simulink model "main_RI_LIEKF_GNSSOutrage"  (R2023a)
settings: Solver=FixedStepAuto  StartTime=0.0  StopTime=220  FixedStep=0.01  RelTol=1e-3
InitFcn:
  | initNavigation0612_AOA;
values from neighbouring files (symbols this model uses):
  CF_enable = 0    [initNavigation.m]
  dt = 0.01    [initNavigation.m]
  dtDelay = -0.03    [initNavigation.m]
  g0 = 9.795    [initNavigation.m]
  gam0_rad = 0/57.3    (= 0)    [initNavigation.m]
  GNSSoutragetime = 90    [initNavigation.m]
  H_sensor_type = 0    [initNavigation.m]
  KF_enable = 1    [initNavigation.m]
  P0 = diag([1*ones(3,1);0.01*ones(3,1);0.1*ones(3,1);0.001*ones(3,1);0.00001*ones(3,1)])    [initNavigation.m]
  P0_RIEKF = diag([1*ones(3,1);0.01*ones(3,1);0.1*ones(3,1);0.001*ones(3,1);0.00001*ones(3,1);      0.01*ones(3,1);[0;2;2]/57.3;[0.1;0.1;0.1]])^2    [initNavigation.m]
  pd0 = 0    [initNavigation.m]
  pe0 = 0    [initNavigation.m]
  phi0_rad = 0/57.3    (= 0)    [initNavigation.m]
  pn0 = 0    [initNavigation.m]
  psi = -178    [initNavigation.m]
  psi0_rad = 0/57.3    (= 0)    [initNavigation.m]
  state_dim = 24    [initNavigation.m]
  Time = 0:0.01:(size(traindata.AttackAngle,1) - 1)*0.01    [NNLiftCoefficientFit.m]
  vd0 = 0    [initNavigation.m]
  ve0 = 0    [initNavigation.m]
  vn0 = 0    [initNavigation.m]
undefined symbols (not defined in the file or in its folder): DiscIntNeverNeededParam, Discrete, INS_CONST, INS_EXPORT, INS_PARAM, magnitude, p, param, pInitialization, sys
libraries: simulink_extras x94, simulink x82, dspstat3 x70, sharedtransform x60, ctrlSharedLib x36, sharedTrackingLibrary x22, matrix_library x15, FMT_Model_Lib x13, deeplib x8, dspsolvers x4, vrlib x4, aerolibconvert2 x1
(part 17 of 28)

== system main_RI_LIEKF_GNSSOutrage/State estimation/LI EKF2/INS propogation/vel//pos update/vel update ==
  dtheta : Inport
  QGC_init : Inport  Port=2
  An : Inport  Port=3
  KFState_dv : Inport  Port=4
  v0 : Inport  Port=5
  Cbn : Inport  Port=6
  Add : Sum
  Delay : Delay  DelayLength=1  InitialConditionSource=Input port  ExternalReset=Rising
      settings: InputPortMap=u0,r5,p4
  Gain : Gain  Gain=dt
  MATLAB Function : MATLAB Function  TreatAsAtomicUnit=on
  Reshape : Reshape  OutputDimensionality=Column vector (2-D)
  vel_k : Outport
  wires:
  Cbn/1 -> MATLAB Function/4(Cbn)
  QGC_init/1 -> Delay/2
  Reshape/1 -> Delay/3
  An/1 -> Gain/1
  v0/1 -> Reshape/1
  Gain/1 -> Add/1
  Delay/1 -> Add/2
  KFState_dv/1 -> MATLAB Function/2(KFState_dv)
  dtheta/1 -> MATLAB Function/1(dtheta)
  Add/1 -> MATLAB Function/3(vel)
  MATLAB Function/1(vel_correct) -> Delay/1, vel_k/1

== system main_RI_LIEKF_GNSSOutrage/State estimation/RI EKF_AOA_LSTM/Error State Kalman Filter/Extended Kalman Filter1/Correct1 ==
  yMeas : Inport  SampleTime=SampleTime
  R : Inport  Port=2  SampleTime=SampleTime
  uMeas : Inport  Port=3  SampleTime=SampleTime
  uBlockOrdering : Inport  Port=4  SampleTime=SampleTime
  Enable : EnablePort
  Correct : MATLAB Function  TreatAsAtomicUnit=on
  Data Store ReadP : DataStoreRead  DataStoreName=P  IndexOptions=Index vector (dialog)  Indices=1  OutputSizes=1
  Data Store ReadX : DataStoreRead  DataStoreName=x  IndexOptions=Index vector (dialog)  Indices=1  OutputSizes=1
  Data Store WriteP : DataStoreWrite  DataStoreName=P  IndexOptions=Index vector (dialog)  Indices=1  OutputSizes=1
  Data Store WriteX : DataStoreWrite  DataStoreName=x  IndexOptions=Index vector (dialog)  Indices=1  OutputSizes=1
  IGG_check : Subsystem  Commented=on
  R1 : InportShadow  Port=2  SampleTime=SampleTime
  RegisterSimulinkFcn : S-Function  FunctionName=ekfukfRegisterSimulinkFcn  Parameters=int32(3), 1, pM.HasAdditiveNoise, SampleTime, DataType, SLFcnsToRegister  SFunctionDeploymentMode=off  EnableBusSupport=off
  Scope : Scope
  Scope1 : Scope
  Scope2 : Scope
  yMeas1 : InportShadow  SampleTime=SampleTime
  yBlockOrdering : Outport  VectorParamsAs1DForOutWhenUnconnected=off
  wires:
  uMeas/1 -> Correct/5(uMeas)
  uBlockOrdering/1 -> Correct/6("blockOrdering ")
  Correct/3(blockOrdering) -> yBlockOrdering/1
  Correct/1(xNew) -> Data Store WriteX/1
  R/1 -> RegisterSimulinkFcn/3, Correct/4(R)
  yMeas/1 -> Scope/1, RegisterSimulinkFcn/2, Correct/3(yMeas)
  Correct/2(P) -> Data Store WriteP/1
  Data Store ReadP/1 -> IGG_check/1(Pk/k_1), Correct/2("P ")
  yMeas1/1 -> IGG_check/2(yMeas)
  R1/1 -> IGG_check/4(R)
  IGG_check/2(w) -> Scope1/1
  Data Store ReadX/1 -> IGG_check/3(X), Correct/1(x), RegisterSimulinkFcn/1
  IGG_check/3(inno) -> Scope2/1

== system main_RI_LIEKF_GNSSOutrage/State estimation/RI EKF_AOA_LSTM/Error State Kalman Filter/Extended Kalman Filter1/Output ==
  uBlockOrdering : Inport
  Data Store Read : DataStoreRead  DataStoreName=x  IndexOptions=Index vector (dialog)  Indices=1  OutputSizes=1
  Data Store Read1 : DataStoreRead  DataStoreName=P  IndexOptions=Index vector (dialog)  Indices=1  OutputSizes=1
  MATLAB Function : MATLAB Function  TreatAsAtomicUnit=on
  x : Outport  VectorParamsAs1DForOutWhenUnconnected=off
  P : Outport  Port=2  VectorParamsAs1DForOutWhenUnconnected=off
  yBlockOrdering : Outport  Port=3  VectorParamsAs1DForOutWhenUnconnected=off
  wires:
  MATLAB Function/1(P) -> P/1
  uBlockOrdering/1 -> yBlockOrdering/1
  Data Store Read1/1 -> MATLAB Function/1(S)
  Data Store Read/1 -> x/1

== system main_RI_LIEKF_GNSSOutrage/State estimation/RI EKF_AOA_LSTM/Error State Kalman Filter/Extended Kalman Filter1/Predict ==
  Q : Inport  SampleTime=SampleTime
  uState : Inport  Port=2  SampleTime=SampleTime
  uBlockOrdering : Inport  Port=3  SampleTime=SampleTime
  Data Store Read1 : DataStoreRead  Commented=on  DataStoreName=feedback_flag_18dim  IndexOptions=Index vector (dialog)  Indices=1  OutputSizes=1
  Data Store Write : DataStoreWrite  DataStoreName=P  IndexOptions=Index vector (dialog)  Indices=1  OutputSizes=1
  Data Store Write1 : DataStoreWrite  DataStoreName=x  IndexOptions=Index vector (dialog)  Indices=1  OutputSizes=1
  Data Store WriteX : DataStoreWrite  DataStoreName=x  IndexOptions=Index vector (dialog)  Indices=1  OutputSizes=1
  Data Store ReadP : DataStoreRead  DataStoreName=P  IndexOptions=Index vector (dialog)  Indices=1  OutputSizes=1
  Data Store ReadX : DataStoreRead  DataStoreName=x  IndexOptions=Index vector (dialog)  Indices=1  OutputSizes=1
  If : If  Commented=on  IfExpression=u1 == 1  ShowElse=off
  If Action Subsystem : Subsystem  Commented=on  TreatAsAtomicUnit=on
  Predict : MATLAB Function  TreatAsAtomicUnit=on
  RegisterSimulinkFcn : S-Function  FunctionName=ekfukfRegisterSimulinkFcn  Parameters=int32(2), 0, pS.HasAdditiveNoise, SampleTime, DataType, SLFcnsToRegister  SFunctionDeploymentMode=off  EnableBusSupport=off
  Zero : Constant  Value=zeros(state_dim,1)  OutDataTypeStr=Inherit: Inherit via back propagation
  wires:
  Zero/1 -> Data Store Write1/1
  If/1 -> If Action Subsystem/Action
  Data Store Read1/1 -> If/1
  uState/1 -> Predict/4(uState)
  uBlockOrdering/1 -> Predict/5(unused)
  Data Store ReadX/1 -> RegisterSimulinkFcn/1, Predict/1(x)
  Predict/1(xNew) -> Data Store WriteX/1
  Q/1 -> RegisterSimulinkFcn/2, Predict/3(Q)
  Predict/2(P) -> Data Store Write/1
  Data Store ReadP/1 -> Predict/2("P ")

== system main_RI_LIEKF_GNSSOutrage/State estimation/RI EKF_AOA_LSTM/Error State Kalman Filter/Simulink Function - State Transition/Cal Phi ==
  Rbn : Inport
  vn : Inport  Port=2
  pn : Inport  Port=3
  Constant : Constant  Value=dt
  MATLAB Function1 : MATLAB Function  TreatAsAtomicUnit=on
  Reshape : Reshape  OutputDimensionality=Column vector (2-D)
  Reshape1 : Reshape  OutputDimensionality=Column vector (2-D)
  Phi : Outport
  wires:
  Constant/1 -> MATLAB Function1/4(dt)
  MATLAB Function1/1(Phi) -> Phi/1
  Rbn/1 -> MATLAB Function1/3(Rbn)
  vn/1 -> Reshape/1
  pn/1 -> Reshape1/1
  Reshape/1 -> MATLAB Function1/1(vn)
  Reshape1/1 -> MATLAB Function1/2(pn)

== system main_RI_LIEKF_GNSSOutrage/State estimation/RI EKF_AOA_LSTM/Error State Kalman Filter/Simulink Function - State Transition1/Cal Phi ==
  Rbn : Inport
  vn : Inport  Port=2
  pn : Inport  Port=3
  Constant : Constant  Value=dt  OutDataTypeStr=single
  MATLAB Function1 : MATLAB Function  TreatAsAtomicUnit=on
  Reshape : Reshape  OutputDimensionality=Column vector (2-D)
  Reshape1 : Reshape  OutputDimensionality=Column vector (2-D)
  Phi : Outport
  wires:
  Reshape1/1 -> MATLAB Function1/2(pn)
  Reshape/1 -> MATLAB Function1/1(vn)
  pn/1 -> Reshape1/1
  vn/1 -> Reshape/1
  Rbn/1 -> MATLAB Function1/3(Rbn)
  MATLAB Function1/1(Phi) -> Phi/1
  Constant/1 -> MATLAB Function1/4(dt)

== system main_RI_LIEKF_GNSSOutrage/State estimation/RI EKF_AOA_LSTM/Error State Kalman Filter/bak/Simulink Function - GPS Measurements1 ==
  DCM_b_n : Inport
  DynamicMeasurementFcn_Dyn : TriggerPort  TriggerType=function-call  IsSimulinkFunction=on  FunctionName=DynamicMeasurementFcn_Dyn  VariantControl=Variant
  Add : Sum  Commented=on
  Add1 : Sum
  Constant : Constant  Commented=on  Value=dt  OutDataTypeStr=single
  Constant6 : Constant  Value=[zeros(3,3),eye(3),zeros(3,12);zeros(3,15),eye(3)]  OutDataTypeStr=single
  Data Type Conversion6 : DataTypeConversion  Commented=on  OutDataTypeStr=single  SaturateOnIntegerOverflow=off  RndMeth=Floor
  From7 : From  Commented=on  GotoTag=DCM_b_n
  Goto : Goto  Commented=on  GotoTag=DCM_b_n
  MATLAB Function1 : MATLAB Function  Commented=on  TreatAsAtomicUnit=on
  Product : Product  Commented=on  Multiplication=Matrix(*)
  Product1 : Product  Multiplication=Matrix(*)
  x : ArgIn  DisableCoverage=on  OutDataTypeStr=single  PortDimensions=18  ArgumentName=x
  v : ArgIn  DisableCoverage=on  Port=2  OutDataTypeStr=single  PortDimensions=6  ArgumentName=v
  y : ArgOut  DisableCoverage=on  OutDataTypeStr=single  PortDimensions=6  ArgumentName=y
  wires:
  Product/1 -> Add/1
  MATLAB Function1/1(H) -> Data Type Conversion6/1
  From7/1 -> MATLAB Function1/1(Cbn)
  Constant/1 -> MATLAB Function1/2(dt)
  DCM_b_n/1 -> Goto/1
  Data Type Conversion6/1 -> Product/1
  Add1/1 -> y/1
  v/1 -> Add1/2
  Product1/1 -> Add1/1
  Constant6/1 -> Product1/1
  x/1 -> Product1/2

== system main_RI_LIEKF_GNSSOutrage/State estimation/RI EKF_AOA_LSTM/Error State Kalman Filter/bak/Simulink Function - GPS Measurements2 ==
  ZUPTMeasurementFcn2 : TriggerPort  TriggerType=function-call  IsSimulinkFunction=on  FunctionName=ZUPTMeasurementFcn2  VariantControl=Variant
  Add : Sum
  Constant6 : Constant  Value=[zeros(3,3),eye(3),zeros(3,12)]  OutDataTypeStr=single
  Product : Product  Multiplication=Matrix(*)
  x : ArgIn  DisableCoverage=on  OutDataTypeStr=single  PortDimensions=18  ArgumentName=x
  v : ArgIn  DisableCoverage=on  Port=2  OutDataTypeStr=single  PortDimensions=3  ArgumentName=v
  y : ArgOut  DisableCoverage=on  OutDataTypeStr=single  PortDimensions=3  ArgumentName=y
  wires:
  Add/1 -> y/1
  Product/1 -> Add/1
  x/1 -> Product/2
  Constant6/1 -> Product/1
  v/1 -> Add/2

== system main_RI_LIEKF_GNSSOutrage/State estimation/RI EKF_AOA_LSTM/Error State Kalman Filter/bak/Simulink Function - State Transition Jacobian ==
  DCM_b_n : Inport
  vn : Inport  Port=2
  pn : Inport  Port=3
  stateTransitionJacobianFcn_Dyn : TriggerPort  TriggerType=function-call  IsSimulinkFunction=on  FunctionName=stateTransitionJacobianFcn_Dyn  VariantControl=Variant
  Cal Phi1 : Subsystem
  Constant : Constant  Value=0.01  OutDataTypeStr=single
  Data Type Conversion1 : DataTypeConversion  OutDataTypeStr=single  SaturateOnIntegerOverflow=off  RndMeth=Floor
  Data Type Conversion6 : DataTypeConversion  OutDataTypeStr=single  SaturateOnIntegerOverflow=off  RndMeth=Floor
  MATLAB Function1 : MATLAB Function  TreatAsAtomicUnit=on
  Product : Product  Multiplication=Matrix(*)
  Terminator : Terminator
  Terminator1 : Terminator
  Transpose : Math  Operator=transpose
  x : ArgIn  DisableCoverage=on  OutDataTypeStr=single  PortDimensions=15  ArgumentName=x
  w : ArgIn  Port=2  OutDataTypeStr=single  PortDimensions=12  ArgumentName=w
  A : ArgOut  DisableCoverage=on  OutDataTypeStr=single  PortDimensions=[15 15]  ArgumentName=A
  G : ArgOut  Port=2  OutDataTypeStr=single  PortDimensions=[15 12]  ArgumentName=G
  wires:
  MATLAB Function1/1(G) -> Data Type Conversion1/1
  x/1 -> Terminator/1
  w/1 -> Terminator1/1
  Cal Phi1/1(Phi) -> Data Type Conversion6/1
  DCM_b_n/1 -> [DCM_b_n]
  pn/1 -> [pn]
  vn/1 -> [vn]
  [vn] -> Cal Phi1/2(vn)
  [pn] -> Cal Phi1/3(pn)
  [DCM_b_n] -> Cal Phi1/1(Rbn)
  [DCM_b_n] -> Transpose/1
  Transpose/1 -> MATLAB Function1/1(Rbn)
  Constant/1 -> MATLAB Function1/4(dt)
  Data Type Conversion6/1 -> Product/1, A/1
  [vn] -> MATLAB Function1/2(vn)
  [pn] -> MATLAB Function1/3(pn)
  Product/1 -> G/1
  Data Type Conversion1/1 -> Product/2

== system main_RI_LIEKF_GNSSOutrage/State estimation/RI EKF_AOA_LSTM/INS propogation/AOA//SA//Vwind update/Subsystem ==
  Cbn : Inport
  vel_NED : Inport  Port=2
  vel_wind_NED : Inport  Port=3
  gyro_raw : Inport  Port=4
  dtheta_a : Inport  Port=5
  elevator_aileron_rudder_deg : Inport  Port=6
  accl_raw : Inport  Port=7
  TAS : Inport  Port=8
  vel_NED_gps : Inport  Port=9
  Enable : EnablePort
  Add : Sum
  Add1 : Sum
  Atan1 : Trigonometry  Operator=atan2
  Atan2 : Trigonometry  Operator=atan2
  Constant : Constant  Value=0  OutDataTypeStr=single
  Data Type Conversion{,1..3} (4 alike) : DataTypeConversion  OutDataTypeStr=single  SaturateOnIntegerOverflow=off  RndMeth=Floor
  Demux : Demux  Outputs=3
  Demux1 : Demux  Outputs=3
  Gain : Gain  Gain=-1
  MATLAB Function : MATLAB Function  TreatAsAtomicUnit=on
  MATLAB Function2 : MATLAB Function  TreatAsAtomicUnit=on
  Mux : Mux  Inputs=2
  Mux1 : Mux  Inputs=2
  Mux2 : Mux  Inputs=2
  Product : Product  Multiplication=Matrix(*)
  Product1 : Product  Multiplication=Matrix(*)
  Rate Transition1 : RateTransition  OutPortSampleTime=dt
  Rate Transition2 : RateTransition  OutPortSampleTime=dt
  Step : Step  Time=GNSSoutragetime-10  OutDataTypeStr=single  SampleTime=0.01
  Step1 : Step  Time=GNSSoutragetime  OutDataTypeStr=single  SampleTime=0.01
  Subsystem : Subsystem
  Subsystem1 : Subsystem
  Subsystem2 : Subsystem
  Switch : Switch  Criteria=u2 > Threshold  SaturateOnIntegerOverflow=off  InputSameDT=off
  Terminator : Terminator
  Terminator1 : Terminator
  Terminator2 : Terminator
  Transpose : Math  Operator=transpose
  Transpose1 : Math  Operator=transpose
  Zero-Order Hold : ZeroOrderHold  SampleTime=0.1
  INSstate_Rab : Outport
  AOA_ref : Outport  Port=2
  SA_ref : Outport  Port=3
  wires:
  Cbn/1 -> Transpose1/1, Transpose/1
  Demux/2 -> Subsystem/2(v), Terminator/1  "v"
  Constant/1 -> Mux2/1
  Demux/1 -> Atan2/2  "u"
  Transpose/1 -> Product/1
  Mux2/1 -> MATLAB Function/1(u)
  Demux/3 -> Atan2/1  "w"
  Add/1 -> Product/2
  Data Type Conversion2/1 -> MATLAB Function2/2(Rbn)  "INSstate_Rab"
  vel_NED/1 -> Add/1
  dtheta_a/1 -> Zero-Order Hold/1
  MATLAB Function/1(Rab) -> Data Type Conversion2/1  "INSstate_Rab"
  Data Type Conversion/1 -> INSstate_Rab/1
  Data Type Conversion1/1 -> Subsystem/1(In1), Demux/1
  Gain/1 -> MATLAB Function2/1(delta)
  Zero-Order Hold/1 -> Gain/1
  Product/1 -> Data Type Conversion1/1
  vel_wind_NED/1 -> Terminator1/1
  gyro_raw/1 -> Subsystem1/1(gyro_raw)
  elevator_aileron_rudder_deg/1 -> Subsystem1/2(elevator_aileron_rudder_deg)
  accl_raw/1 -> Subsystem1/3(accl_raw)  "az"
  TAS/1 -> Subsystem1/4(TAS)
  Step/1 -> Rate Transition1/1
  Rate Transition1/1 -> Subsystem1/Enable
  Mux/1 -> Switch/1
  Subsystem1/1(AOA_LSTM_rad out) -> Mux/1
  Subsystem1/2(SA_LSTM_rad) -> Mux/2
  Atan2/1 -> Mux1/1  "alpha"
  Subsystem/1(beta) -> Mux1/2
  Mux1/1 -> Switch/3
  Switch/1 -> Mux2/2
  MATLAB Function2/1(Rbn_correct) -> Data Type Conversion/1  "INSstate_Rab"
  Product1/1 -> Data Type Conversion3/1
  Data Type Conversion3/1 -> Demux1/1, Subsystem2/1(In1)
  vel_NED_gps/1 -> Add1/1
  Add1/1 -> Product1/2
  Demux1/3 -> Atan1/1  "w"
  Transpose1/1 -> Product1/1
  Demux1/1 -> Atan1/2  "u"
  Demux1/2 -> Terminator2/1, Subsystem2/2(v)  "v"
  Atan1/1 -> AOA_ref/1  "alpha"
  Subsystem2/1(beta) -> SA_ref/1
  Step1/1 -> Rate Transition2/1
  Rate Transition2/1 -> Switch/2

== system main_RI_LIEKF_GNSSOutrage/State estimation/RI EKF_AOA_LSTM/INS propogation/AOA//SA//Vwind update/Subsystem1 ==
  vel_NED : Inport
  Compare To Constant : simulink/Logic and Bit Operations/Compare To Constant  relop=>=  const=10  OutDataTypeStr=boolean
  Math Function : Math  Operator=magnitude^2
  Sqrt : Sqrt
  Sum of Elements : Sum  Inputs=+
  AOA_Estimation_flag : Outport
  wires:
  Sum of Elements/1 -> Sqrt/1
  Sqrt/1 -> Compare To Constant/1
  Compare To Constant/1 -> AOA_Estimation_flag/1
  Math Function/1 -> Sum of Elements/1
  vel_NED/1 -> Math Function/1

== system main_RI_LIEKF_GNSSOutrage/State estimation/RI EKF_AOA_LSTM/INS propogation/AOA//SA//Vwind update/Subsystem2 ==
  Rbn : Inport
  INSstate_Rab : Inport  Port=2
  INSstate_v : Inport  Port=3
  TAS : Inport  Port=4
  dv_wind : Inport  Port=5
  Enable : EnablePort
  Add : Sum  Inputs=+-+
  Atan2 : Trigonometry  Operator=atan2
  Compare To Constant : simulink/Logic and Bit Operations/Compare To Constant  relop=>=  const=0.5  OutDataTypeStr=boolean
  Demux : Demux  Outputs=3
  Math Function : Math  Operator=magnitude^2
  Memory : Memory
  Product : Product  Inputs=3  Multiplication=Matrix(*)
  Radians to Degrees : simulink_extras/Transformations/Radians to Degrees
  Scope : Scope  NumInputPorts=2
  Scope1 : Scope
  Sqrt : Sqrt
  Sum of Elements : Sum  Inputs=+
  Switch : Switch  Criteria=u2 > Threshold  SaturateOnIntegerOverflow=off  InputSameDT=off
  Zero-Order Hold : ZeroOrderHold  SampleTime=0.1
  v_wind_out : Outport
  wires:
  dv_wind/1 -> Zero-Order Hold/1
  Demux/1 -> Atan2/1
  Demux/2 -> Atan2/2
  Product/1 -> Add/2
  Atan2/1 -> Radians to Degrees/1
  Radians to Degrees/1 -> Memory/1, Scope1/1, Switch/1
  INSstate_v/1 -> Add/1
  TAS/1 -> Product/3
  INSstate_Rab/1 -> Product/2
  Rbn/1 -> Product/1
  Zero-Order Hold/1 -> Add/3, Scope/2
  Sqrt/1 -> Compare To Constant/1
  Sum of Elements/1 -> Sqrt/1
  Math Function/1 -> Sum of Elements/1
  Add/1 -> v_wind_out/1, Scope/1, Math Function/1, Demux/1
  Compare To Constant/1 -> Switch/2
  Memory/1 -> Switch/3

== system main_RI_LIEKF_GNSSOutrage/State estimation/RI EKF_AOA_LSTM/INS propogation/Init_PVQ/Horizontal_attitude ==
  note: fai
  note: gamma
  accl_mean_B_m/s_LPF : Inport  PortDimensions=3
  Magn_mean_B_guess_LPF : Inport  Port=2
  Enable : EnablePort
  Add : Sum  Inputs=+-
  Add1 : Sum
  Add2 : Sum
  Asin : Trigonometry  Operator=asin
  Atan2 : Trigonometry  Operator=atan2
  Data Type Conversion : DataTypeConversion  SaturateOnIntegerOverflow=off  RndMeth=Floor
  Deal with zero : Subsystem
  Degrees to Radians : simulink_extras/Transformations/Degrees to Radians
  Degrees to Radians1 : simulink_extras/Transformations/Degrees to Radians
  Demux : Demux  Outputs=3
  Display : Display
  Divide : Product  Inputs=*/  OutDataTypeStr=single
  Gain1 : Gain  Gain=-1
  Gain2 : Gain  Gain=-1
  Magnetic declination : Constant  Value=param.fusion.magDeclDeg  OutDataTypeStr=single
  Magnetic declination1 : Constant  Value=param.control.MagnheadingCorrection  OutDataTypeStr=uint8
  Math Function : Math  Operator=magnitude^2  SignedPower=on
  Mux : Mux  Inputs=3
  Mux1 : Mux  Inputs=3
  Mux3 : Mux  Inputs=3
  Product : Product  Multiplication=Matrix(*)
  Quaternions to Direction Cosine Matrix : sharedtransform/Quaternions to  Direction Cosine Matrix  aMode=aMode
  Radians to Degrees : simulink_extras/Transformations/Radians to Degrees
  Rotation Angles to Quaternions : sharedtransform/Rotation Angles to Quaternions  rotationOrder=ZYX  aMode=aMode
  Rotation Angles to Quaternions1 : sharedtransform/Rotation Angles to Quaternions  rotationOrder=ZYX  aMode=aMode
  Scope : Scope
  Scope1 : Scope
  Selector : Selector  InputPortWidth=3  IndexOptions=Index vector (dialog)  Indices=[2]  OutputSizes=1
  Selector1 : Selector  InputPortWidth=3  IndexOptions=Index vector (dialog)  Indices=[1]  OutputSizes=1
  Sqrt : Sqrt
  Sum of Elements : Sum  Inputs=+
  Switch : Switch  Threshold=0.5  SaturateOnIntegerOverflow=off  InputSameDT=off
  Terminator : Terminator
  Transpose : Math  Operator=transpose  SignedPower=on
  Trigonometric Function1 : Trigonometry  Operator=atan2
  phi0_rad : Constant  Value=phi0_rad  OutDataTypeStr=single
  phi0_rad1 : Constant  Value=gam0_rad  OutDataTypeStr=single
  psi_zero : Constant  Value=psi  OutDataTypeStr=single
  psi_zero1 : Constant  Commented=on  Value=psi  OutDataTypeStr=single
  quat_0 : Outport  PortDimensions=4
  wires:
  accl_mean_B_m/s_LPF/1 -> Demux/1
  Sqrt/1 -> Deal with zero/1(In1)
  Deal with zero/1(Out1) -> Divide/2
  Trigonometric Function1/1 -> Gain2/1
  Demux/1 -> Divide/1, Mux/2
  Demux/2 -> Mux/1, Trigonometric Function1/1
  Demux/3 -> Gain1/1
  Sum of Elements/1 -> Sqrt/1
  Divide/1 -> Asin/1
  Mux/1 -> Math Function/1
  Math Function/1 -> Sum of Elements/1
  Mux1/1 -> Rotation Angles to Quaternions/1
  psi_zero/1 -> Degrees to Radians1/1
  Add1/1 -> Mux3/2, Mux1/2
  Add2/1 -> Mux3/3, Mux1/3
  Rotation Angles to Quaternions/1 -> Switch/3, Switch/1, Quaternions to Direction Cosine Matrix/1  "q0_no_yaw"
  Quaternions to Direction Cosine Matrix/1 -> Transpose/1
  Magn_mean_B_guess_LPF/1 -> Product/2
  Product/1 -> Selector/1, Selector1/1  "magNED"
  Selector1/1 -> Atan2/2  "magN"
  Selector/1 -> Atan2/1  "magE"
  Atan2/1 -> Add/2
  Magnetic declination/1 -> Degrees to Radians/1
  Add/1 -> Radians to Degrees/1, Mux3/1  "psi_calbymag"
  Mux3/1 -> Rotation Angles to Quaternions1/1
  Transpose/1 -> Product/1
  Gain1/1 -> Trigonometric Function1/2, Mux/3
  Degrees to Radians1/1 -> Mux1/1
  Degrees to Radians/1 -> Terminator/1
  Magnetic declination1/1 -> Data Type Conversion/1, Switch/2
  Switch/1 -> Scope1/1, quat_0/1
  Data Type Conversion/1 -> Scope/1
  Radians to Degrees/1 -> Display/1
  Asin/1 -> Add1/2
  phi0_rad/1 -> Add1/1
  phi0_rad1/1 -> Add2/1
  Gain2/1 -> Add2/2

== system main_RI_LIEKF_GNSSOutrage/State estimation/RI EKF_AOA_LSTM/INS propogation/Init_PVQ/Subsystem ==
  data : Inport
  Buffer : Buffer  N=50  V=49  OutputFrames=off
  Buffer1 : Buffer  N=50  V=49  OutputFrames=off
  Buffer2 : Buffer  N=50  V=49  ic=-g0  OutputFrames=off
  Demux : Demux  Outputs=3
  Mean4 : dspstat3/Mean  run=off  reset_popup=None  directionMode=Entire input  dimension=3  roiEnable=off  roiType=Rectangles  roiPortion=Entire ROI  roiOutput=Individual statistics for each ROI  roiFlag=off  roundingMode=Floor  overflowMode=off  outputDataTypeStr=Inherit: Same as accumulator  outputMin=[]  outputMax=[]  outputLastDataTypeStr=Inherit: Same as accumulator
  Mean5 : dspstat3/Mean  run=off  reset_popup=None  directionMode=Entire input  dimension=3  roiEnable=off  roiType=Rectangles  roiPortion=Entire ROI  roiOutput=Individual statistics for each ROI  roiFlag=off  roundingMode=Floor  overflowMode=off  outputDataTypeStr=Inherit: Same as accumulator  outputMin=[]  outputMax=[]  outputLastDataTypeStr=Inherit: Same as accumulator
  Mean6 : dspstat3/Mean  run=off  reset_popup=None  directionMode=Entire input  dimension=3  roiEnable=off  roiType=Rectangles  roiPortion=Entire ROI  roiOutput=Individual statistics for each ROI  roiFlag=off  roundingMode=Floor  overflowMode=off  outputDataTypeStr=Inherit: Same as accumulator  outputMin=[]  outputMax=[]  outputLastDataTypeStr=Inherit: Same as accumulator
  Scope : Scope  NumInputPorts=2
  Vector Concatenate : Concatenate  NumInputs=3
  mean_data : Outport
  wires:
  Mean6/1 -> Vector Concatenate/3
  Demux/2 -> Buffer1/1
  Buffer/1 -> Mean4/1  "fbx_buff"
  Mean5/1 -> Vector Concatenate/2
  Buffer2/1 -> Mean6/1  "fbz_buff"
  Demux/1 -> Buffer/1
  Buffer1/1 -> Mean5/1  "fby_buff"
  Demux/3 -> Buffer2/1
  Mean4/1 -> Vector Concatenate/1
  Vector Concatenate/1 -> Scope/2, mean_data/1
  data/1 -> Scope/1, Demux/1

== system main_RI_LIEKF_GNSSOutrage/State estimation/RI EKF_AOA_LSTM/INS propogation/Init_PVQ/Subsystem1 ==
  data : Inport
  Buffer : Buffer  N=50  V=49  OutputFrames=off
  Buffer1 : Buffer  N=50  V=49  OutputFrames=off
  Buffer2 : Buffer  N=50  V=49  OutputFrames=off
  Demux : Demux  Outputs=3
  Mean4 : dspstat3/Mean  run=off  reset_popup=None  directionMode=Entire input  dimension=3  roiEnable=off  roiType=Rectangles  roiPortion=Entire ROI  roiOutput=Individual statistics for each ROI  roiFlag=off  roundingMode=Floor  overflowMode=off  outputDataTypeStr=Inherit: Same as accumulator  outputMin=[]  outputMax=[]  outputLastDataTypeStr=Inherit: Same as accumulator
  Mean5 : dspstat3/Mean  run=off  reset_popup=None  directionMode=Entire input  dimension=3  roiEnable=off  roiType=Rectangles  roiPortion=Entire ROI  roiOutput=Individual statistics for each ROI  roiFlag=off  roundingMode=Floor  overflowMode=off  outputDataTypeStr=Inherit: Same as accumulator  outputMin=[]  outputMax=[]  outputLastDataTypeStr=Inherit: Same as accumulator
  Mean6 : dspstat3/Mean  run=off  reset_popup=None  directionMode=Entire input  dimension=3  roiEnable=off  roiType=Rectangles  roiPortion=Entire ROI  roiOutput=Individual statistics for each ROI  roiFlag=off  roundingMode=Floor  overflowMode=off  outputDataTypeStr=Inherit: Same as accumulator  outputMin=[]  outputMax=[]  outputLastDataTypeStr=Inherit: Same as accumulator
  Vector Concatenate : Concatenate  NumInputs=3
  mean_data : Outport
  wires:
  data/1 -> Demux/1
  Vector Concatenate/1 -> mean_data/1
  Mean4/1 -> Vector Concatenate/1
  Demux/3 -> Buffer2/1
  Buffer1/1 -> Mean5/1  "fby_buff"
  Demux/1 -> Buffer/1
  Buffer2/1 -> Mean6/1  "fbz_buff"
  Mean5/1 -> Vector Concatenate/2
  Buffer/1 -> Mean4/1  "fbx_buff"
  Demux/2 -> Buffer1/1
  Mean6/1 -> Vector Concatenate/3

== system main_RI_LIEKF_GNSSOutrage/State estimation/RI EKF_AOA_LSTM/INS propogation/accl bias compensation/error compensation1 ==
  dda : Inport
  QGC_init : Inport  Port=2
  Add3 : Sum
  Delay : Delay  DelayLength=1  InitialCondition=zeros(3,1)  ExternalReset=Level hold
      settings: InputPortMap=u0,r5
  da : Outport
  wires:
  Delay/1 -> Add3/2
  dda/1 -> Add3/1
  QGC_init/1 -> Delay/2
  Add3/1 -> da/1, Delay/1

== system main_RI_LIEKF_GNSSOutrage/State estimation/RI EKF_AOA_LSTM/INS propogation/accl bias compensation1/error compensation1 ==
  dda : Inport
  QGC_init : Inport  Port=2
  Add3 : Sum
  Delay : Delay  DelayLength=1  InitialCondition=zeros(3,1)  ExternalReset=Level hold
      settings: InputPortMap=u0,r5
  da : Outport
  wires:
  Add3/1 -> Delay/1, da/1
  QGC_init/1 -> Delay/2
  dda/1 -> Add3/1
  Delay/1 -> Add3/2

== system main_RI_LIEKF_GNSSOutrage/State estimation/RI EKF_AOA_LSTM/INS propogation/accl bias compensation2/error compensation1 ==
  dda : Inport
  QGC_init : Inport  Port=2
  Add3 : Sum
  Delay : Delay  DelayLength=1  InitialCondition=zeros(3,1)  ExternalReset=Level hold
      settings: InputPortMap=u0,r5
  da : Outport
  wires:
  Delay/1 -> Add3/2
  dda/1 -> Add3/1
  QGC_init/1 -> Delay/2
  Add3/1 -> da/1, Delay/1

== system main_RI_LIEKF_GNSSOutrage/State estimation/RI EKF_AOA_LSTM/INS propogation/gyro bias compensation/error compensation ==
  ddg : Inport
  Enable : Inport  Port=2
  QGC_init : Inport  Port=3
  Add3 : Sum
  Delay : Delay  DelayLength=1  InitialCondition=zeros(3,1)  ExternalReset=Level hold
      settings: InputPortMap=u0,r5
  If Action Subsystem1 : Subsystem  TreatAsAtomicUnit=on
  If1 : If  IfExpression=u1 == 1  ShowElse=off
  Scope : Scope
  dg : Outport
  wires:
  Enable/1 -> Scope/1, If1/1
  If1/1 -> If Action Subsystem1/Action
  Delay/1 -> Add3/2
  Add3/1 -> Delay/1, dg/1
  ddg/1 -> Add3/1
  QGC_init/1 -> Delay/2

== system main_RI_LIEKF_GNSSOutrage/State estimation/RI EKF_AOA_LSTM/INS propogation/vel//pos update/Kinematic Equation ==
  Cbn : Inport
  Ab : Inport  Port=2
  Add : Sum  Inputs=+-
  Add1 : Sum  Inputs=+-
  Constant : Constant  Value=[0 0 -g0]  OutDataTypeStr=single
  Constant1 : Constant  Value=[0 0 -g0]  OutDataTypeStr=single
  Product : Product  Multiplication=Matrix(*)  RndMeth=Zero
  Product1 : Product  Multiplication=Matrix(*)  RndMeth=Zero
  Scope : Scope
  Scope1 : Scope  NumInputPorts=2
  Transpose : Math  Operator=transpose
  An : Outport
  ab_nog : Outport  Port=2
  wires:
  Cbn/1 -> Transpose/1, Product/1
  Add/1 -> An/1, Scope1/2
  Ab/1 -> Product/2, Add1/1, Scope1/1
  Product/1 -> Scope/1, Add/1
  Constant/1 -> Add/2
  Transpose/1 -> Product1/1  "Cnb"
  Constant1/1 -> Product1/2  "gn"
  Product1/1 -> Add1/2  "gb"
  Add1/1 -> ab_nog/1  "ab_nog"

== system main_RI_LIEKF_GNSSOutrage/State estimation/RI EKF_AOA_LSTM/INS propogation/vel//pos update/pos update ==
  dtheta : Inport
  vel_k : Inport  Port=2
  dp : Inport  Port=3
  QGC_init : Inport  Port=4
  p0 : Inport  Port=5
  Add1 : Sum
  Delay1 : Delay  DelayLength=1  InitialConditionSource=Input port  ExternalReset=Rising
      settings: InputPortMap=u0,r5,p4
  Gain1 : Gain  Gain=dt
  MATLAB Function : MATLAB Function  TreatAsAtomicUnit=on
  Reshape1 : Reshape  OutputDimensionality=Column vector (2-D)
  p_k : Outport
  wires:
  p0/1 -> Reshape1/1
  QGC_init/1 -> Delay1/2
  Reshape1/1 -> Delay1/3
  Delay1/1 -> Add1/2
  Gain1/1 -> Add1/1
  vel_k/1 -> Gain1/1
  dtheta/1 -> MATLAB Function/1(dtheta)
  dp/1 -> MATLAB Function/2(KFState_dp)
  Add1/1 -> MATLAB Function/3(pos)
  MATLAB Function/1(pos_correct) -> Delay1/1, p_k/1

== system main_RI_LIEKF_GNSSOutrage/State estimation/RI EKF_AOA_LSTM/INS propogation/vel//pos update/vel update ==
  dtheta : Inport
  QGC_init : Inport  Port=2
  An : Inport  Port=3
  KFState_dv : Inport  Port=4
  v0 : Inport  Port=5
  Add : Sum
  Delay : Delay  DelayLength=1  InitialConditionSource=Input port  ExternalReset=Rising
      settings: InputPortMap=u0,r5,p4
  Gain : Gain  Gain=dt
  MATLAB Function : MATLAB Function  TreatAsAtomicUnit=on
  Reshape : Reshape  OutputDimensionality=Column vector (2-D)
  vel_k : Outport
  wires:
  QGC_init/1 -> Delay/2
  Reshape/1 -> Delay/3
  An/1 -> Gain/1
  v0/1 -> Reshape/1
  Gain/1 -> Add/1
  Delay/1 -> Add/2
  KFState_dv/1 -> MATLAB Function/2(KFState_dv)
  dtheta/1 -> MATLAB Function/1(dtheta)
  Add/1 -> MATLAB Function/3(vel)
  MATLAB Function/1(vel_correct) -> Delay/1, vel_k/1

== system main_RI_LIEKF_GNSSOutrage/State estimation/RI EKF_AOA_direct/Error State Kalman Filter/Extended Kalman Filter1/Correct1 ==
  yMeas : Inport  SampleTime=SampleTime
  R : Inport  Port=2  SampleTime=SampleTime
  uMeas : Inport  Port=3  SampleTime=SampleTime
  uBlockOrdering : Inport  Port=4  SampleTime=SampleTime
  Enable : EnablePort
  Correct : MATLAB Function  TreatAsAtomicUnit=on
  Data Store ReadP : DataStoreRead  DataStoreName=P  IndexOptions=Index vector (dialog)  Indices=1  OutputSizes=1
  Data Store ReadX : DataStoreRead  DataStoreName=x  IndexOptions=Index vector (dialog)  Indices=1  OutputSizes=1
  Data Store WriteP : DataStoreWrite  DataStoreName=P  IndexOptions=Index vector (dialog)  Indices=1  OutputSizes=1
  Data Store WriteX : DataStoreWrite  DataStoreName=x  IndexOptions=Index vector (dialog)  Indices=1  OutputSizes=1
  IGG_check : Subsystem  Commented=on
  R1 : InportShadow  Port=2  SampleTime=SampleTime
  RegisterSimulinkFcn : S-Function  FunctionName=ekfukfRegisterSimulinkFcn  Parameters=int32(3), 1, pM.HasAdditiveNoise, SampleTime, DataType, SLFcnsToRegister  SFunctionDeploymentMode=off  EnableBusSupport=off
  Scope : Scope
  Scope1 : Scope
  Scope2 : Scope
  yMeas1 : InportShadow  SampleTime=SampleTime
  yBlockOrdering : Outport  VectorParamsAs1DForOutWhenUnconnected=off
  wires:
  IGG_check/3(inno) -> Scope2/1
  Data Store ReadX/1 -> RegisterSimulinkFcn/1, Correct/1(x), IGG_check/3(X)
  IGG_check/2(w) -> Scope1/1
  R1/1 -> IGG_check/4(R)
  yMeas1/1 -> IGG_check/2(yMeas)
  Data Store ReadP/1 -> Correct/2("P "), IGG_check/1(Pk/k_1)
  Correct/2(P) -> Data Store WriteP/1
  yMeas/1 -> Correct/3(yMeas), RegisterSimulinkFcn/2, Scope/1
  R/1 -> Correct/4(R), RegisterSimulinkFcn/3
  Correct/1(xNew) -> Data Store WriteX/1
  Correct/3(blockOrdering) -> yBlockOrdering/1
  uBlockOrdering/1 -> Correct/6("blockOrdering ")
  uMeas/1 -> Correct/5(uMeas)

== system main_RI_LIEKF_GNSSOutrage/State estimation/RI EKF_AOA_direct/Error State Kalman Filter/Extended Kalman Filter1/Output ==
  uBlockOrdering : Inport
  Data Store Read : DataStoreRead  DataStoreName=x  IndexOptions=Index vector (dialog)  Indices=1  OutputSizes=1
  Data Store Read1 : DataStoreRead  DataStoreName=P  IndexOptions=Index vector (dialog)  Indices=1  OutputSizes=1
  MATLAB Function : MATLAB Function  TreatAsAtomicUnit=on
  x : Outport  VectorParamsAs1DForOutWhenUnconnected=off
  P : Outport  Port=2  VectorParamsAs1DForOutWhenUnconnected=off
  yBlockOrdering : Outport  Port=3  VectorParamsAs1DForOutWhenUnconnected=off
  wires:
  Data Store Read/1 -> x/1
  Data Store Read1/1 -> MATLAB Function/1(S)
  uBlockOrdering/1 -> yBlockOrdering/1
  MATLAB Function/1(P) -> P/1

== system main_RI_LIEKF_GNSSOutrage/State estimation/RI EKF_AOA_direct/Error State Kalman Filter/Extended Kalman Filter1/Predict ==
  Q : Inport  SampleTime=SampleTime
  uState : Inport  Port=2  SampleTime=SampleTime
  uBlockOrdering : Inport  Port=3  SampleTime=SampleTime
  Data Store Read1 : DataStoreRead  Commented=on  DataStoreName=feedback_flag_18dim  IndexOptions=Index vector (dialog)  Indices=1  OutputSizes=1
  Data Store Write : DataStoreWrite  DataStoreName=P  IndexOptions=Index vector (dialog)  Indices=1  OutputSizes=1
  Data Store Write1 : DataStoreWrite  DataStoreName=x  IndexOptions=Index vector (dialog)  Indices=1  OutputSizes=1
  Data Store WriteX : DataStoreWrite  DataStoreName=x  IndexOptions=Index vector (dialog)  Indices=1  OutputSizes=1
  Data Store ReadP : DataStoreRead  DataStoreName=P  IndexOptions=Index vector (dialog)  Indices=1  OutputSizes=1
  Data Store ReadX : DataStoreRead  DataStoreName=x  IndexOptions=Index vector (dialog)  Indices=1  OutputSizes=1
  If : If  Commented=on  IfExpression=u1 == 1  ShowElse=off
  If Action Subsystem : Subsystem  Commented=on  TreatAsAtomicUnit=on
  Predict : MATLAB Function  TreatAsAtomicUnit=on
  RegisterSimulinkFcn : S-Function  FunctionName=ekfukfRegisterSimulinkFcn  Parameters=int32(2), 0, pS.HasAdditiveNoise, SampleTime, DataType, SLFcnsToRegister  SFunctionDeploymentMode=off  EnableBusSupport=off
  Zero : Constant  Value=zeros(state_dim,1)  OutDataTypeStr=Inherit: Inherit via back propagation
  wires:
  Data Store ReadP/1 -> Predict/2("P ")
  Predict/2(P) -> Data Store Write/1
  Q/1 -> Predict/3(Q), RegisterSimulinkFcn/2
  Predict/1(xNew) -> Data Store WriteX/1
  Data Store ReadX/1 -> Predict/1(x), RegisterSimulinkFcn/1
  uBlockOrdering/1 -> Predict/5(unused)
  uState/1 -> Predict/4(uState)
  Data Store Read1/1 -> If/1
  If/1 -> If Action Subsystem/Action
  Zero/1 -> Data Store Write1/1

== system main_RI_LIEKF_GNSSOutrage/State estimation/RI EKF_AOA_direct/Error State Kalman Filter/Simulink Function - State Transition/Cal Phi ==
  Rbn : Inport
  vn : Inport  Port=2
  pn : Inport  Port=3
  Constant : Constant  Value=dt
  MATLAB Function1 : MATLAB Function  TreatAsAtomicUnit=on
  Reshape : Reshape  OutputDimensionality=Column vector (2-D)
  Reshape1 : Reshape  OutputDimensionality=Column vector (2-D)
  Phi : Outport
  wires:
  Reshape1/1 -> MATLAB Function1/2(pn)
  Reshape/1 -> MATLAB Function1/1(vn)
  pn/1 -> Reshape1/1
  vn/1 -> Reshape/1
  Rbn/1 -> MATLAB Function1/3(Rbn)
  MATLAB Function1/1(Phi) -> Phi/1
  Constant/1 -> MATLAB Function1/4(dt)

== system main_RI_LIEKF_GNSSOutrage/State estimation/RI EKF_AOA_direct/Error State Kalman Filter/Simulink Function - State Transition1/Cal Phi ==
  Rbn : Inport
  vn : Inport  Port=2
  pn : Inport  Port=3
  Constant : Constant  Value=dt  OutDataTypeStr=single
  MATLAB Function1 : MATLAB Function  TreatAsAtomicUnit=on
  Reshape : Reshape  OutputDimensionality=Column vector (2-D)
  Reshape1 : Reshape  OutputDimensionality=Column vector (2-D)
  Phi : Outport
  wires:
  Constant/1 -> MATLAB Function1/4(dt)
  MATLAB Function1/1(Phi) -> Phi/1
  Rbn/1 -> MATLAB Function1/3(Rbn)
  vn/1 -> Reshape/1
  pn/1 -> Reshape1/1
  Reshape/1 -> MATLAB Function1/1(vn)
  Reshape1/1 -> MATLAB Function1/2(pn)

== system main_RI_LIEKF_GNSSOutrage/State estimation/RI EKF_AOA_direct/Error State Kalman Filter/bak/Simulink Function - GPS Measurements1 ==
  DCM_b_n : Inport
  DynamicMeasurementFcn_Dyn : TriggerPort  TriggerType=function-call  IsSimulinkFunction=on  FunctionName=DynamicMeasurementFcn_Dyn  VariantControl=Variant
  Add : Sum  Commented=on
  Add1 : Sum
  Constant : Constant  Commented=on  Value=dt  OutDataTypeStr=single
  Constant6 : Constant  Value=[zeros(3,3),eye(3),zeros(3,12);zeros(3,15),eye(3)]  OutDataTypeStr=single
  Data Type Conversion6 : DataTypeConversion  Commented=on  OutDataTypeStr=single  SaturateOnIntegerOverflow=off  RndMeth=Floor
  From7 : From  Commented=on  GotoTag=DCM_b_n
  Goto : Goto  Commented=on  GotoTag=DCM_b_n
  MATLAB Function1 : MATLAB Function  Commented=on  TreatAsAtomicUnit=on
  Product : Product  Commented=on  Multiplication=Matrix(*)
  Product1 : Product  Multiplication=Matrix(*)
  x : ArgIn  DisableCoverage=on  OutDataTypeStr=single  PortDimensions=18  ArgumentName=x
  v : ArgIn  DisableCoverage=on  Port=2  OutDataTypeStr=single  PortDimensions=6  ArgumentName=v
  y : ArgOut  DisableCoverage=on  OutDataTypeStr=single  PortDimensions=6  ArgumentName=y
  wires:
  x/1 -> Product1/2
  Constant6/1 -> Product1/1
  Product1/1 -> Add1/1
  v/1 -> Add1/2
  Add1/1 -> y/1
  Data Type Conversion6/1 -> Product/1
  DCM_b_n/1 -> Goto/1
  Constant/1 -> MATLAB Function1/2(dt)
  From7/1 -> MATLAB Function1/1(Cbn)
  MATLAB Function1/1(H) -> Data Type Conversion6/1
  Product/1 -> Add/1

== system main_RI_LIEKF_GNSSOutrage/State estimation/RI EKF_AOA_direct/Error State Kalman Filter/bak/Simulink Function - GPS Measurements2 ==
  ZUPTMeasurementFcn2 : TriggerPort  TriggerType=function-call  IsSimulinkFunction=on  FunctionName=ZUPTMeasurementFcn2  VariantControl=Variant
  Add : Sum
  Constant6 : Constant  Value=[zeros(3,3),eye(3),zeros(3,12)]  OutDataTypeStr=single
  Product : Product  Multiplication=Matrix(*)
  x : ArgIn  DisableCoverage=on  OutDataTypeStr=single  PortDimensions=18  ArgumentName=x
  v : ArgIn  DisableCoverage=on  Port=2  OutDataTypeStr=single  PortDimensions=3  ArgumentName=v
  y : ArgOut  DisableCoverage=on  OutDataTypeStr=single  PortDimensions=3  ArgumentName=y
  wires:
  v/1 -> Add/2
  Constant6/1 -> Product/1
  x/1 -> Product/2
  Product/1 -> Add/1
  Add/1 -> y/1

== system main_RI_LIEKF_GNSSOutrage/State estimation/RI EKF_AOA_direct/Error State Kalman Filter/bak/Simulink Function - State Transition Jacobian ==
  DCM_b_n : Inport
  vn : Inport  Port=2
  pn : Inport  Port=3
  stateTransitionJacobianFcn_Dyn : TriggerPort  TriggerType=function-call  IsSimulinkFunction=on  FunctionName=stateTransitionJacobianFcn_Dyn  VariantControl=Variant
  Cal Phi1 : Subsystem
  Constant : Constant  Value=0.01  OutDataTypeStr=single
  Data Type Conversion1 : DataTypeConversion  OutDataTypeStr=single  SaturateOnIntegerOverflow=off  RndMeth=Floor
  Data Type Conversion6 : DataTypeConversion  OutDataTypeStr=single  SaturateOnIntegerOverflow=off  RndMeth=Floor
  MATLAB Function1 : MATLAB Function  TreatAsAtomicUnit=on
  Product : Product  Multiplication=Matrix(*)
  Terminator : Terminator
  Terminator1 : Terminator
  Transpose : Math  Operator=transpose
  x : ArgIn  DisableCoverage=on  OutDataTypeStr=single  PortDimensions=15  ArgumentName=x
  w : ArgIn  Port=2  OutDataTypeStr=single  PortDimensions=12  ArgumentName=w
  A : ArgOut  DisableCoverage=on  OutDataTypeStr=single  PortDimensions=[15 15]  ArgumentName=A
  G : ArgOut  Port=2  OutDataTypeStr=single  PortDimensions=[15 12]  ArgumentName=G
  wires:
  Data Type Conversion1/1 -> Product/2
  Product/1 -> G/1
  [pn] -> MATLAB Function1/3(pn)
  [vn] -> MATLAB Function1/2(vn)
  Data Type Conversion6/1 -> A/1, Product/1
  Constant/1 -> MATLAB Function1/4(dt)
  Transpose/1 -> MATLAB Function1/1(Rbn)
  [DCM_b_n] -> Transpose/1
  [DCM_b_n] -> Cal Phi1/1(Rbn)
  [pn] -> Cal Phi1/3(pn)
  [vn] -> Cal Phi1/2(vn)
  vn/1 -> [vn]
  pn/1 -> [pn]
  DCM_b_n/1 -> [DCM_b_n]
  Cal Phi1/1(Phi) -> Data Type Conversion6/1
  w/1 -> Terminator1/1
  x/1 -> Terminator/1
  MATLAB Function1/1(G) -> Data Type Conversion1/1

== system main_RI_LIEKF_GNSSOutrage/State estimation/RI EKF_AOA_direct/INS propogation/AOA//SA//Vwind update/Subsystem ==
  note: Subsystem2
  Cbn : Inport
  vel_NED : Inport  Port=2
  vel_wind_NED : Inport  Port=3
  gyro_raw : Inport  Port=4
  dtheta_a : Inport  Port=5
  elevator_aileron_rudder_deg : Inport  Port=6
  accl_raw : Inport  Port=7
  TAS : Inport  Port=8
  Enable : EnablePort
  Add : Sum  Commented=on
  Atan2 : Trigonometry  Commented=on  Operator=atan2
  Constant : Constant  Value=0  OutDataTypeStr=single
  Constant1 : Constant  Value=0
  Data Type Conversion{,2..4,11} (5 alike) : DataTypeConversion  OutDataTypeStr=single  SaturateOnIntegerOverflow=off  RndMeth=Floor
  Data Type Conversion1 : DataTypeConversion  Commented=on  OutDataTypeStr=single  SaturateOnIntegerOverflow=off  RndMeth=Floor
  Degrees to Radians : simulink_extras/Transformations/Degrees to Radians
  Degrees to Radians1 : simulink_extras/Transformations/Degrees to Radians
  Demux : Demux  Commented=on  Outputs=3
  Demux1 : Demux  Outputs=3
  Direction Cosine Matrix to Rotation Angles : sharedtransform/Direction Cosine Matrix to Rotation Angles  rotationOrder=ZYX  aMode=aMode  action=None  tolerance=eps(2)
      settings: LibrarySourceBlock=|
      | aerolibtransform2/Direction Cosine Matrix
      | to Rotation Angles
  Gain : Gain  Gain=-1
  MATLAB Function : MATLAB Function  TreatAsAtomicUnit=on
  MATLAB Function1 : MATLAB Function  TreatAsAtomicUnit=on
  MATLAB Function2 : MATLAB Function  TreatAsAtomicUnit=on
  Mux : Mux  Commented=on  Inputs=2
  Mux1 : Mux  Inputs=2
  Mux2 : Mux  Inputs=2
  Product : Product  Commented=on  Multiplication=Matrix(*)
  Rate Transition1 : RateTransition  Commented=on  OutPortSampleTime=dt
  Step : Step  Commented=on  Time=GNSSoutragetime  OutDataTypeStr=single  SampleTime=0.01
  Subsystem : Subsystem  Commented=on
  Subsystem1 : Subsystem  Commented=on
  Subsystem3 : Subsystem
  Subsystem4 : Subsystem
  Switch : Switch  Commented=on  Criteria=u2 > Threshold  SaturateOnIntegerOverflow=off  InputSameDT=off
  Switch1 : Switch  Threshold=1  SaturateOnIntegerOverflow=off  InputSameDT=off
  Switch2 : Switch  Threshold=1  SaturateOnIntegerOverflow=off  InputSameDT=off
  Terminator : Terminator  Commented=on
  Terminator1 : Terminator  Commented=on
  Terminator2 : Terminator
  Transpose : Math  Commented=on  Operator=transpose
  Transpose1 : Math  Operator=transpose
  Zero-Order Hold : ZeroOrderHold  SampleTime=0.1
  INSstate_Rab : Outport
  wires:
  MATLAB Function2/1(Rbn_correct) -> Data Type Conversion/1  "INSstate_Rab"
  Mux1/1 -> Mux2/2, Switch/3
  Subsystem1/2(SA_LSTM_rad) -> Mux/2
  Subsystem1/1(AOA_LSTM_rad out) -> Mux/1
  Mux/1 -> Switch/1
  Rate Transition1/1 -> Subsystem1/Enable, Switch/2
  Step/1 -> Rate Transition1/1
  TAS/1 -> Subsystem1/4(TAS)
  accl_raw/1 -> Subsystem1/3(accl_raw)  "az"
  elevator_aileron_rudder_deg/1 -> Subsystem1/2(elevator_aileron_rudder_deg)
  gyro_raw/1 -> Subsystem1/1(gyro_raw)
  vel_wind_NED/1 -> Terminator1/1
  Product/1 -> Data Type Conversion1/1
  Zero-Order Hold/1 -> Gain/1
  Gain/1 -> MATLAB Function2/1(delta)
  Data Type Conversion1/1 -> Demux/1, Subsystem/1(In1)
  Data Type Conversion/1 -> INSstate_Rab/1
  MATLAB Function/1(Rab) -> Data Type Conversion2/1  "INSstate_Rab"
  dtheta_a/1 -> Zero-Order Hold/1
  Data Type Conversion2/1 -> MATLAB Function2/2(Rbn)  "INSstate_Rab"
  Add/1 -> Product/2
  Demux/3 -> Atan2/1  "w"
  Mux2/1 -> MATLAB Function/1(u)
  Transpose/1 -> Product/1
  Demux/1 -> Atan2/2  "u"
  Constant/1 -> Mux2/1
  Demux/2 -> Terminator/1, Subsystem/2(v)  "v"
  Cbn/1 -> Transpose1/1
  Transpose1/1 -> Direction Cosine Matrix to Rotation Angles/1
  Data Type Conversion11/1 -> Demux1/1
  Demux1/3 -> Terminator2/1  "phi_rad"
  Demux1/2 -> Subsystem3/1(RIEKF_att_Deg)  "theta_rad"
  Demux1/1 -> Subsystem3/3(psi_Deg)  "psi_rad"
  Direction Cosine Matrix to Rotation Angles/1 -> Data Type Conversion11/1
  MATLAB Function1/1(y) -> Switch1/1
  Switch1/1 -> Data Type Conversion4/1  "INSstate_Rab"
  Data Type Conversion4/1 -> Degrees to Radians1/1
  Subsystem3/2(SA_direct_Deg) -> MATLAB Function1/1(dpsi)
  Switch2/1 -> Data Type Conversion3/1  "INSstate_Rab"
  Subsystem4/1(AOA_Estimation_flag) -> Switch1/2, Switch2/2, Subsystem3/Enable
  Constant1/1 -> Switch1/3, Switch2/3
  Data Type Conversion3/1 -> Degrees to Radians/1
  vel_NED/1 -> Subsystem4/1(vel_NED), Subsystem3/2(vel_NED)
  Subsystem3/1(AOA_direct_Deg) -> Switch2/1
  Degrees to Radians/1 -> Mux1/1
  Degrees to Radians1/1 -> Mux1/2

== system main_RI_LIEKF_GNSSOutrage/State estimation/RI EKF_AOA_direct/INS propogation/AOA//SA//Vwind update/Subsystem1 ==
  vel_NED : Inport
  Compare To Constant : simulink/Logic and Bit Operations/Compare To Constant  relop=>=  const=10  OutDataTypeStr=boolean
  Math Function : Math  Operator=magnitude^2
  Sqrt : Sqrt
  Sum of Elements : Sum  Inputs=+
  AOA_Estimation_flag : Outport
  wires:
  vel_NED/1 -> Math Function/1
  Math Function/1 -> Sum of Elements/1
  Compare To Constant/1 -> AOA_Estimation_flag/1
  Sqrt/1 -> Compare To Constant/1
  Sum of Elements/1 -> Sqrt/1

== system main_RI_LIEKF_GNSSOutrage/State estimation/RI EKF_AOA_direct/INS propogation/AOA//SA//Vwind update/Subsystem2 ==
  Rbn : Inport
  INSstate_Rab : Inport  Port=2
  INSstate_v : Inport  Port=3
  TAS : Inport  Port=4
  dv_wind : Inport  Port=5
  Enable : EnablePort
  Add : Sum  Inputs=+-+
  Atan2 : Trigonometry  Operator=atan2
  Compare To Constant : simulink/Logic and Bit Operations/Compare To Constant  relop=>=  const=0.5  OutDataTypeStr=boolean
  Demux : Demux  Outputs=3
  Math Function : Math  Operator=magnitude^2
  Memory : Memory
  Product : Product  Inputs=3  Multiplication=Matrix(*)
  Radians to Degrees : simulink_extras/Transformations/Radians to Degrees
  Scope : Scope  NumInputPorts=2
  Scope1 : Scope
  Sqrt : Sqrt
  Sum of Elements : Sum  Inputs=+
  Switch : Switch  Criteria=u2 > Threshold  SaturateOnIntegerOverflow=off  InputSameDT=off
  Zero-Order Hold : ZeroOrderHold  SampleTime=0.1
  v_wind_out : Outport
  wires:
  Memory/1 -> Switch/3
  Compare To Constant/1 -> Switch/2
  Add/1 -> Demux/1, Math Function/1, Scope/1, v_wind_out/1
  Math Function/1 -> Sum of Elements/1
  Sum of Elements/1 -> Sqrt/1
  Sqrt/1 -> Compare To Constant/1
  Zero-Order Hold/1 -> Scope/2, Add/3
  Rbn/1 -> Product/1
  INSstate_Rab/1 -> Product/2
  TAS/1 -> Product/3
  INSstate_v/1 -> Add/1
  Radians to Degrees/1 -> Switch/1, Scope1/1, Memory/1
  Atan2/1 -> Radians to Degrees/1
  Product/1 -> Add/2
  Demux/2 -> Atan2/2
  Demux/1 -> Atan2/1
  dv_wind/1 -> Zero-Order Hold/1
